simulink model "kalman_at_20_hz"  (R2013b)
settings: Solver=FixedStepDiscrete  StartTime=10  StopTime=250  FixedStep=0.05  RelTol=1e-3
settings Model: Creator=Franta  LastModifiedBy=Franta

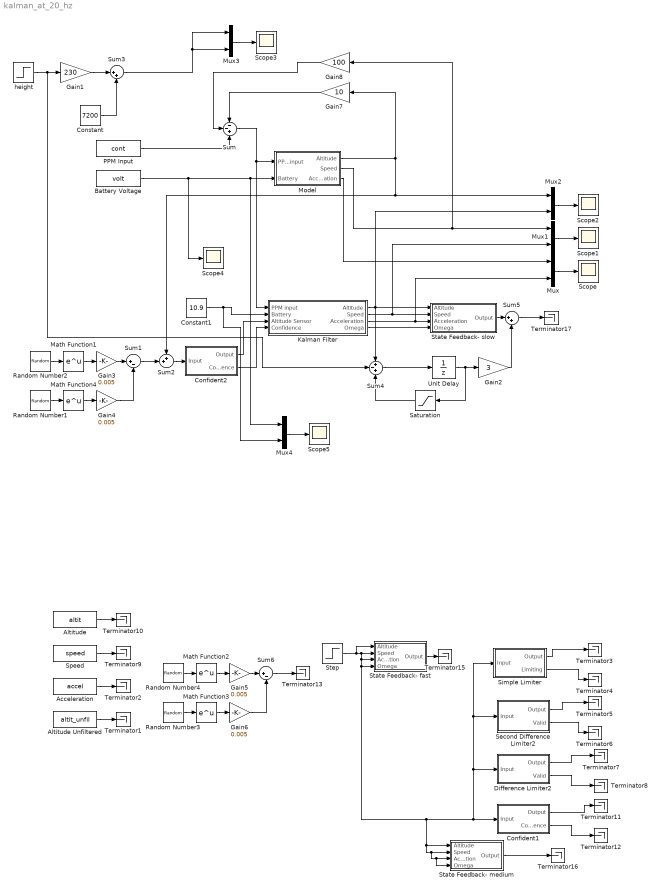
== system kalman_at_20_hz ==
  Acceleration : FromWorkspace  VariableName=accel  SampleTime=0  OutputAfterFinalValue=Holding final value
  Altitude : FromWorkspace  VariableName=altit  SampleTime=0  OutputAfterFinalValue=Holding final value
  Altitude Unfiltered : FromWorkspace  VariableName=altit_unfil  SampleTime=0  OutputAfterFinalValue=Holding final value
  Battery Voltage : FromWorkspace  VariableName=volt  SampleTime=0  OutputAfterFinalValue=Holding final value
  Confident1 : Subsystem
  Confident2 : Subsystem
  Constant : Constant  Value=7200
  Constant1 : Constant  Value=10.9
  Difference Limiter2 : Subsystem
  Gain1 : Gain  Gain=230
  Gain2 : Gain  Gain=3
  Gain{3..6} (4 alike) : Gain  Gain=0.005
  Gain7 : Gain  Gain=10
  Gain8 : Gain  Gain=100
  Kalman Filter : Subsystem
  Math Function{1..4} (4 alike) : Math  SaturateOnIntegerOverflow=on
  Model : Subsystem
  Mux{,1..4} (5 alike) : Mux  Inputs=2
  PPM Input : FromWorkspace  VariableName=cont  SampleTime=0  OutputAfterFinalValue=Holding final value
  Random Number1 : RandomNumber  Variance=4  Seed=1  SampleTime=0.05
  Random Number2 : RandomNumber  Variance=4  SampleTime=0.05
  Random Number3 : RandomNumber  Variance=4  Seed=1  SampleTime=0.05
  Random Number4 : RandomNumber  Variance=4  SampleTime=0.05
  Saturation : Saturate  UpperLimit=100  LowerLimit=-100
  Scope{,1..5} (6 alike) : Scope
      Scope settings: YMin=0  YMax=47.5
      Scope1 settings: TimeRange=50
      Scope2 settings: SaveName=ScopeData2
      Scope3 settings: SaveName=ScopeData3
      Scope4 settings: SaveName=ScopeData4
      Scope5 settings: SaveName=ScopeData5
  Second Difference Limiter2 : Subsystem
  Simple Limiter : Subsystem
  Speed : FromWorkspace  VariableName=speed  SampleTime=0  OutputAfterFinalValue=Holding final value
  State Feedback- fast : Subsystem
  State Feedback- medium : Subsystem
  State Feedback- slow : Subsystem
  Step : Step  Time=150  SampleTime=0
  Sum : Sum  Inputs=--+
  Sum1 : Sum  Inputs=|+-
  Sum2 : Sum  Inputs=++|
  Sum3 : Sum  Inputs=|++
  Sum4 : Sum  Inputs=+-+
  Sum5 : Sum  Inputs=|++
  Sum6 : Sum  Inputs=|+-
  Terminator{1..13,15..17} (16 alike) : Terminator
  Unit Delay : UnitDelay  SampleTime=-1
  height : Step  Time=225  SampleTime=0
  wires:
  Mux/1 -> Scope/1
  Mux1/1 -> Scope1/1
  Mux2/1 -> Scope2/1
  Battery Voltage/1 -> Scope4/1, Mux4/1, Model/2(Battery)
  Kalman Filter/3(Acceleration) -> Mux/2, State Feedback- slow/3(Acceleration)
  Simple Limiter/1(Output) -> Terminator3/1
  Simple Limiter/2(Limiting) -> Terminator4/1
  Second Difference Limiter2/1(Output) -> Terminator5/1
  Second Difference Limiter2/2(Valid) -> Terminator6/1
  Difference Limiter2/1(Output) -> Terminator7/1
  Difference Limiter2/2(Valid) -> Terminator8/1
  Kalman Filter/1(Altitude) -> Mux2/2, State Feedback- slow/1(Altitude), Sum4/1
  Kalman Filter/2(Speed) -> Mux1/2, State Feedback- slow/2(Speed)
  Confident1/1(Output) -> Terminator11/1
  Confident1/2(Confidence) -> Terminator12/1
  Confident2/1(Output) -> Kalman Filter/3(Altitude Sensor)
  Confident2/2(Confidence) -> Kalman Filter/4(Confidence)
  Mux3/1 -> Scope3/1
  height/1 -> Sum4/2, Gain1/1
  Gain1/1 -> Sum3/1
  Constant/1 -> Sum3/2
  Step/1 -> State Feedback- fast/3(Acceleration), State Feedback- fast/4(Omega), State Feedback- medium/4(Omega), State Feedback- medium/3(Acceleration), State Feedback- medium/2(Speed), State Feedback- medium/1(Altitude), Simple Limiter/1(Input), Second Difference Limiter2/1(Input), Difference Limiter2/1(Input), Confident1/1(Input), State Feedback- fast/2(Speed), State Feedback- fast/1(Altitude)
  Sum4/1 -> Unit Delay/1
  State Feedback- medium/1(Output) -> Terminator16/1
  Unit Delay/1 -> Gain2/1, Saturation/1
  Gain2/1 -> Sum5/2
  State Feedback- slow/1(Output) -> Sum5/1
  State Feedback- fast/1(Output) -> Terminator15/1
  Kalman Filter/4(Omega) -> State Feedback- slow/4(Omega)
  Model/1(Altitude) -> Gain7/1, Mux2/1, Sum2/1
  Model/2(Speed) -> Gain8/1, Mux1/1
  Model/3(Acceleration) -> Mux/1
  Altitude Unfiltered/1 -> Terminator1/1
  Sum2/1 -> Confident2/1(Input)
  Sum1/1 -> Sum2/2
  Random Number4/1 -> Math Function2/1
  Math Function2/1 -> Gain5/1
  Random Number3/1 -> Math Function3/1
  Math Function3/1 -> Gain6/1
  Gain6/1 -> Sum6/2
  Gain5/1 -> Sum6/1
  Sum6/1 -> Terminator13/1
  Acceleration/1 -> Terminator2/1
  Speed/1 -> Terminator9/1
  Altitude/1 -> Terminator10/1
  Random Number2/1 -> Math Function1/1
  Math Function1/1 -> Gain3/1
  Random Number1/1 -> Math Function4/1
  Math Function4/1 -> Gain4/1
  Gain4/1 -> Sum1/2
  Gain3/1 -> Sum1/1
  Saturation/1 -> Sum4/3
  Sum5/1 -> Terminator17/1
  Sum3/1 -> Mux3/2, Mux3/1
  Sum/1 -> Kalman Filter/1(PPM input), Model/1(PPM input)
  Gain7/1 -> Sum/1
  PPM Input/1 -> Sum/3
  Gain8/1 -> Sum/2
  Constant1/1 -> Mux4/2, Kalman Filter/2(Battery)
  Mux4/1 -> Scope5/1

== system kalman_at_20_hz/Confident1 ==
  Input : Inport
  MATLAB Function : MATLAB Function  TreatAsAtomicUnit=on
  Threshold : Constant  Value=0.35
  Unit Delay : UnitDelay  InitialCondition=0.5  SampleTime=-1
  Unit Delay1 : UnitDelay  SampleTime=-1
  Output : Outport
  Confidence : Outport  Port=2
  wires:
  Unit Delay1/1 -> MATLAB Function/4(cycles)
  MATLAB Function/3(cyclesBlind) -> Unit Delay1/1
  MATLAB Function/2(confidence) -> Confidence/1
  Unit Delay/1 -> MATLAB Function/3(lastGood)
  MATLAB Function/1(good) -> Unit Delay/1
  Threshold/1 -> MATLAB Function/2(threshold)
  Input/1 -> MATLAB Function/1(input), Output/1

== system kalman_at_20_hz/Confident2 ==
  Input : Inport
  MATLAB Function : MATLAB Function  TreatAsAtomicUnit=on
  Threshold : Constant  Value=0.35
  Unit Delay : UnitDelay  InitialCondition=0.5  SampleTime=-1
  Unit Delay1 : UnitDelay  SampleTime=-1
  Output : Outport
  Confidence : Outport  Port=2
  wires:
  Input/1 -> Output/1, MATLAB Function/1(input)
  Threshold/1 -> MATLAB Function/2(threshold)
  MATLAB Function/1(good) -> Unit Delay/1
  Unit Delay/1 -> MATLAB Function/3(lastGood)
  MATLAB Function/2(confidence) -> Confidence/1
  MATLAB Function/3(cyclesBlind) -> Unit Delay1/1
  Unit Delay1/1 -> MATLAB Function/4(cycles)

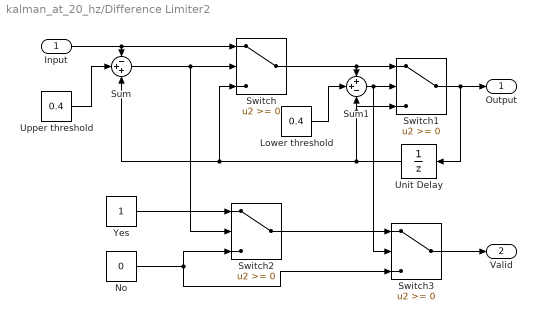
== system kalman_at_20_hz/Difference Limiter2 ==
  Input : Inport
  Lower threshold : Constant  Value=0.4
  No : Constant  Value=0
  Sum : Sum  Inputs=-++
  Sum1 : Sum  Inputs=++-
  Switch{,1..3} (4 alike) : Switch
  Unit Delay : UnitDelay  InitialCondition=1  SampleTime=-1
  Upper threshold : Constant  Value=0.4
  Yes : Constant
  Output : Outport
  Valid : Outport  Port=2
  wires:
  Lower threshold/1 -> Sum1/2
  Switch/1 -> Switch1/1, Sum1/1
  Switch1/1 -> Unit Delay/1, Output/1
  Upper threshold/1 -> Sum/2
  Input/1 -> Switch/1, Sum/1
  Unit Delay/1 -> Sum/3, Switch/3, Switch1/3, Sum1/3
  Sum/1 -> Switch2/2, Switch/2
  Sum1/1 -> Switch3/2, Switch1/2
  Yes/1 -> Switch2/1
  No/1 -> Switch2/3, Switch3/3
  Switch2/1 -> Switch3/1
  Switch3/1 -> Valid/1

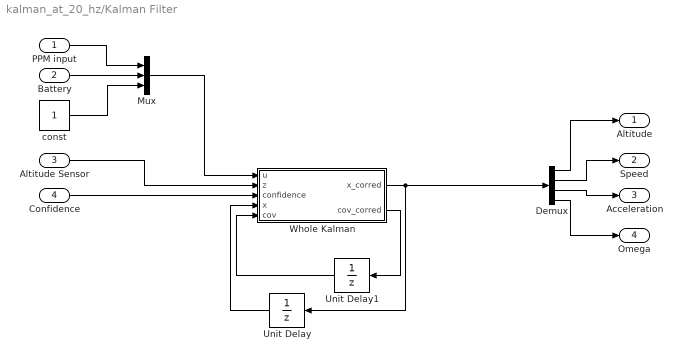
== system kalman_at_20_hz/Kalman Filter ==
  PPM input : Inport
  Battery : Inport  Port=2
  Altitude Sensor : Inport  Port=3
  Confidence : Inport  Port=4
  Demux : Demux
  Mux : Mux  Inputs=3
  Unit Delay : UnitDelay  InitialCondition=[0 0 0 0]'  SampleTime=-1
  Unit Delay1 : UnitDelay  InitialCondition=[1 0 0 0; 0 1 0 0; 0 0 1 0; 0 0 0 1]  SampleTime=-1
  Whole Kalman : MATLAB Function  TreatAsAtomicUnit=on
  const : Constant
  Altitude : Outport
  Speed : Outport  Port=2
  Acceleration : Outport  Port=3
  Omega : Outport  Port=4
  wires:
  Whole Kalman/1(x_corred) -> Demux/1, Unit Delay/1
  Mux/1 -> Whole Kalman/1(u)
  PPM input/1 -> Mux/1
  Battery/1 -> Mux/2
  const/1 -> Mux/3
  Demux/2 -> Speed/1
  Demux/3 -> Acceleration/1
  Demux/1 -> Altitude/1
  Demux/4 -> Omega/1
  Unit Delay1/1 -> Whole Kalman/5(cov)
  Whole Kalman/2(cov_corred) -> Unit Delay1/1
  Unit Delay/1 -> Whole Kalman/4(x)
  Confidence/1 -> Whole Kalman/3(confidence)
  Altitude Sensor/1 -> Whole Kalman/2(z)

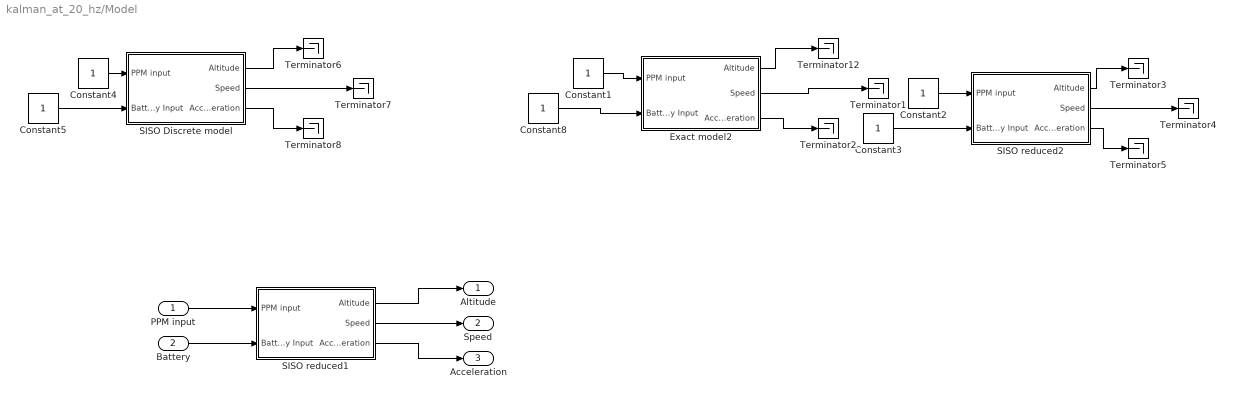
== system kalman_at_20_hz/Model ==
  PPM input : Inport
  Battery : Inport  Port=2
  Constant{1..5,8} (6 alike) : Constant
  Exact model2 : Subsystem
  SISO Discrete model : Subsystem
  SISO reduced1 : Subsystem
  SISO reduced2 : Subsystem
  Terminator{1..8,12} (9 alike) : Terminator
  Altitude : Outport
  Speed : Outport  Port=2
  Acceleration : Outport  Port=3
  wires:
  SISO reduced2/1(Altitude) -> Terminator3/1
  SISO reduced2/2(Speed) -> Terminator4/1
  SISO reduced2/3(Acceleration) -> Terminator5/1
  Constant3/1 -> SISO reduced2/2(Battery Input)
  Constant2/1 -> SISO reduced2/1(PPM input)
  SISO Discrete model/1(Altitude) -> Terminator6/1
  SISO Discrete model/2(Speed) -> Terminator7/1
  SISO Discrete model/3(Acceleration) -> Terminator8/1
  Constant5/1 -> SISO Discrete model/2(Battery Input)
  Constant4/1 -> SISO Discrete model/1(PPM input)
  Constant8/1 -> Exact model2/2(Battery Input)
  Constant1/1 -> Exact model2/1(PPM input)
  Exact model2/1(Altitude) -> Terminator12/1
  Exact model2/2(Speed) -> Terminator1/1
  Exact model2/3(Acceleration) -> Terminator2/1
  PPM input/1 -> SISO reduced1/1(PPM input)
  Battery/1 -> SISO reduced1/2(Battery Input)
  SISO reduced1/1(Altitude) -> Altitude/1
  SISO reduced1/2(Speed) -> Speed/1
  SISO reduced1/3(Acceleration) -> Acceleration/1

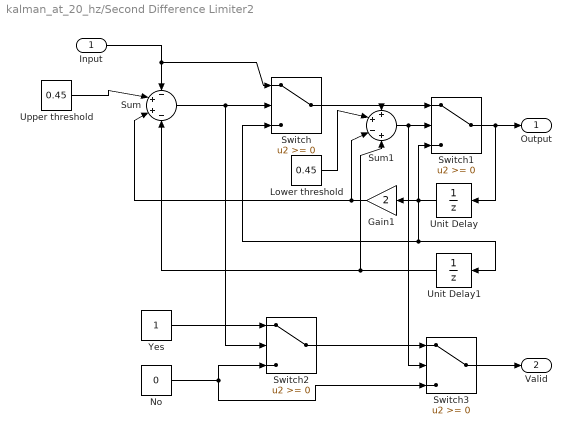
== system kalman_at_20_hz/Second Difference Limiter2 ==
  Input : Inport
  Gain1 : Gain  Gain=2
  Lower threshold : Constant  Value=0.45
  No : Constant  Value=0
  Sum : Sum  Inputs=-++-
  Sum1 : Sum  Inputs=++-+
  Switch{,1..3} (4 alike) : Switch
  Unit Delay : UnitDelay  InitialCondition=1  SampleTime=-1
  Unit Delay1 : UnitDelay  InitialCondition=1  SampleTime=-1
  Upper threshold : Constant  Value=0.45
  Yes : Constant
  Output : Outport
  Valid : Outport  Port=2
  wires:
  Gain1/1 -> Sum1/3, Sum/3
  Switch3/1 -> Valid/1
  Switch2/1 -> Switch3/1
  No/1 -> Switch3/3, Switch2/3
  Yes/1 -> Switch2/1
  Sum1/1 -> Switch1/2, Switch3/2
  Sum/1 -> Switch2/2, Switch/2
  Unit Delay/1 -> Gain1/1, Switch1/3, Unit Delay1/1, Switch/3
  Input/1 -> Switch/1, Sum/1
  Upper threshold/1 -> Sum/2
  Switch1/1 -> Output/1, Unit Delay/1
  Switch/1 -> Switch1/1, Sum1/1
  Lower threshold/1 -> Sum1/2
  Unit Delay1/1 -> Sum1/4, Sum/4

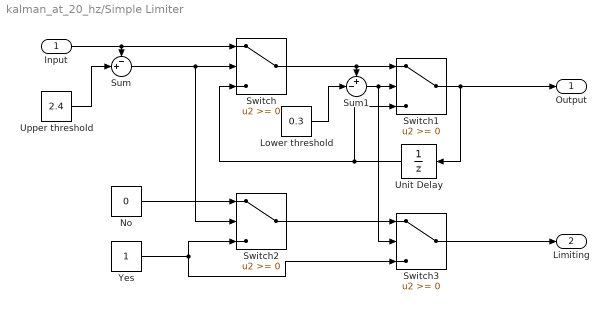
== system kalman_at_20_hz/Simple Limiter ==
  Input : Inport
  Lower threshold : Constant  Value=0.3
  No : Constant  Value=0
  Sum : Sum  Inputs=-+|
  Sum1 : Sum  Inputs=+-|
  Switch{,1..3} (4 alike) : Switch
  Unit Delay : UnitDelay  SampleTime=-1
  Upper threshold : Constant  Value=2.4
  Yes : Constant
  Output : Outport
  Limiting : Outport  Port=2
  wires:
  Unit Delay/1 -> Switch1/3, Switch/3
  Sum/1 -> Switch2/2, Switch/2
  Input/1 -> Sum/1, Switch/1
  Upper threshold/1 -> Sum/2
  Switch1/1 -> Output/1, Unit Delay/1
  Sum1/1 -> Switch3/2, Switch1/2
  Switch/1 -> Sum1/1, Switch1/1
  Lower threshold/1 -> Sum1/2
  No/1 -> Switch2/1
  Yes/1 -> Switch2/3, Switch3/3
  Switch2/1 -> Switch3/1
  Switch3/1 -> Limiting/1

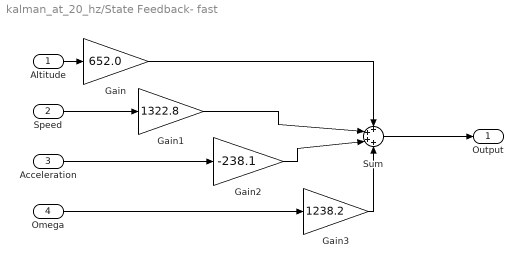
== system kalman_at_20_hz/State Feedback- fast ==
  Altitude : Inport
  Speed : Inport  Port=2
  Acceleration : Inport  Port=3
  Omega : Inport  Port=4
  Gain : Gain  Gain=652.0
  Gain1 : Gain  Gain=1322.8
  Gain2 : Gain  Gain=-238.1
  Gain3 : Gain  Gain=1238.2
  Sum : Sum  Inputs=++++
  Output : Outport
  wires:
  Altitude/1 -> Gain/1
  Speed/1 -> Gain1/1
  Acceleration/1 -> Gain2/1
  Omega/1 -> Gain3/1
  Gain/1 -> Sum/1
  Gain1/1 -> Sum/2
  Gain2/1 -> Sum/3
  Gain3/1 -> Sum/4
  Sum/1 -> Output/1

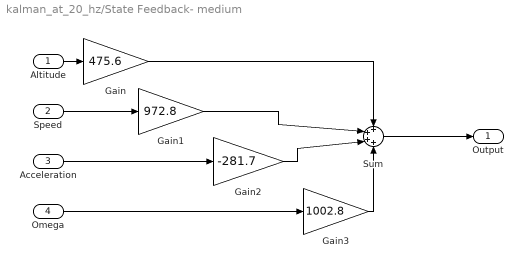
== system kalman_at_20_hz/State Feedback- medium ==
  Altitude : Inport
  Speed : Inport  Port=2
  Acceleration : Inport  Port=3
  Omega : Inport  Port=4
  Gain : Gain  Gain=475.6
  Gain1 : Gain  Gain=972.8
  Gain2 : Gain  Gain=-281.7
  Gain3 : Gain  Gain=1002.8
  Sum : Sum  Inputs=++++
  Output : Outport
  wires:
  Sum/1 -> Output/1
  Gain3/1 -> Sum/4
  Gain2/1 -> Sum/3
  Gain1/1 -> Sum/2
  Gain/1 -> Sum/1
  Omega/1 -> Gain3/1
  Acceleration/1 -> Gain2/1
  Speed/1 -> Gain1/1
  Altitude/1 -> Gain/1

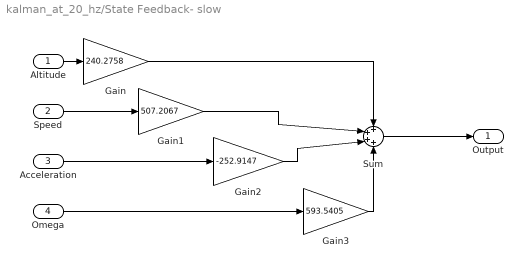
== system kalman_at_20_hz/State Feedback- slow ==
  Altitude : Inport
  Speed : Inport  Port=2
  Acceleration : Inport  Port=3
  Omega : Inport  Port=4
  Gain : Gain  Gain=240.2758
  Gain1 : Gain  Gain=507.2067
  Gain2 : Gain  Gain=-252.9147
  Gain3 : Gain  Gain=593.5405
  Sum : Sum  Inputs=++++
  Output : Outport
  wires:
  Altitude/1 -> Gain/1
  Speed/1 -> Gain1/1
  Acceleration/1 -> Gain2/1
  Omega/1 -> Gain3/1
  Gain/1 -> Sum/1
  Gain1/1 -> Sum/2
  Gain2/1 -> Sum/3
  Gain3/1 -> Sum/4
  Sum/1 -> Output/1

== system kalman_at_20_hz/Model/Exact model2 ==
  PPM input : Inport
  Battery Input : Inport  Port=2
  Demux : Demux
  Discrete State-Space : DiscreteStateSpace  A=[1 0.05 0 0; 0 1 0.05 0; 0 0 0 1; 0 0 -0.65658 1.5714]  B=[0 0 0; 0 0 0; 0.00091141 -0.36830 -2.8005; 0.0011525 -0.052414 -7.5757]  C=[1 0 0 0; 0 1 0 0; 0 0 1 0; 0 0 0 1]  D=[0 0 0; 0 0 0; 0 0 0; 0 0 0]  SampleTime=0.05
  Mux : Mux  Inputs=3
  Terminator : Terminator
  const : Constant
  Altitude : Outport
  Speed : Outport  Port=2
  Acceleration : Outport  Port=3
  wires:
  const/1 -> Mux/3
  Battery Input/1 -> Mux/2
  PPM input/1 -> Mux/1
  Discrete State-Space/1 -> Demux/1
  Demux/3 -> Acceleration/1
  Demux/2 -> Speed/1
  Demux/1 -> Altitude/1
  Mux/1 -> Discrete State-Space/1
  Demux/4 -> Terminator/1

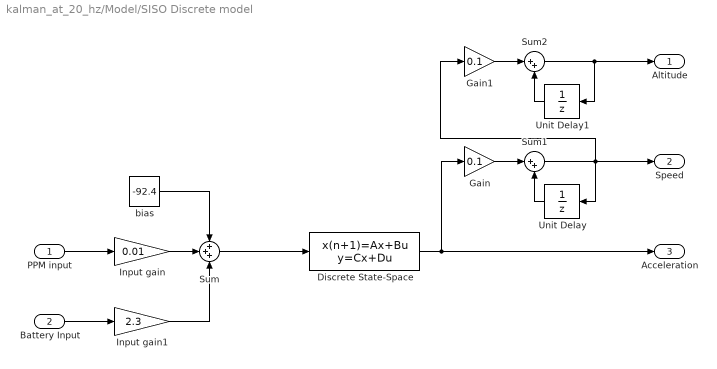
== system kalman_at_20_hz/Model/SISO Discrete model ==
  PPM input : Inport
  Battery Input : Inport  Port=2
  Discrete State-Space : DiscreteStateSpace  A=[0 1; -0.67523 1.64069]  B=[0.28811; 0.18591]  C=[1 0]  D=0  SampleTime=0.1
  Gain : Gain  Gain=0.1
  Gain1 : Gain  Gain=0.1
  Input gain : Gain  Gain=0.01
  Input gain1 : Gain  Gain=2.3
  Sum : Sum  Inputs=+++
  Sum1 : Sum  Inputs=|++
  Sum2 : Sum  Inputs=|++
  Unit Delay : UnitDelay  SampleTime=-1
  Unit Delay1 : UnitDelay  InitialCondition=1  SampleTime=-1
  bias : Constant  Value=-92.4
  Altitude : Outport
  Speed : Outport  Port=2
  Acceleration : Outport  Port=3
  wires:
  PPM input/1 -> Input gain/1
  Battery Input/1 -> Input gain1/1
  Input gain/1 -> Sum/2
  Input gain1/1 -> Sum/3
  bias/1 -> Sum/1
  Sum/1 -> Discrete State-Space/1
  Discrete State-Space/1 -> Gain/1, Acceleration/1
  Unit Delay/1 -> Sum1/2
  Sum1/1 -> Unit Delay/1, Gain1/1, Speed/1
  Sum2/1 -> Unit Delay1/1, Altitude/1
  Unit Delay1/1 -> Sum2/2
  Gain/1 -> Sum1/1
  Gain1/1 -> Sum2/1

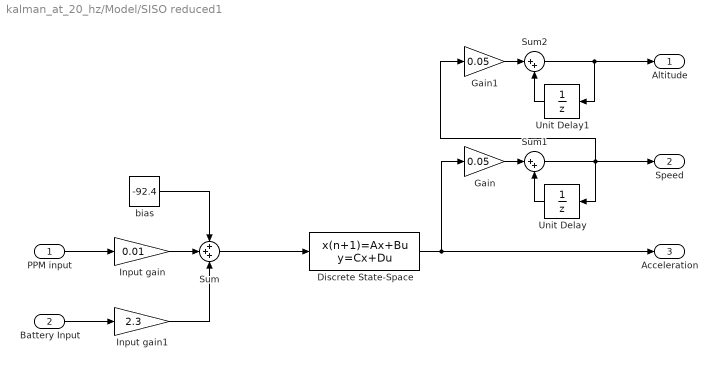
== system kalman_at_20_hz/Model/SISO reduced1 ==
  PPM input : Inport
  Battery Input : Inport  Port=2
  Discrete State-Space : DiscreteStateSpace  A=[0.8379]  B=[0.1382]  C=[1]  D=0  SampleTime=0.05
  Gain : Gain  Gain=0.05
  Gain1 : Gain  Gain=0.05
  Input gain : Gain  Gain=0.01
  Input gain1 : Gain  Gain=2.3
  Sum : Sum  Inputs=+++
  Sum1 : Sum  Inputs=|++
  Sum2 : Sum  Inputs=|++
  Unit Delay : UnitDelay  SampleTime=-1
  Unit Delay1 : UnitDelay  SampleTime=-1
  bias : Constant  Value=-92.4
  Altitude : Outport
  Speed : Outport  Port=2
  Acceleration : Outport  Port=3
  wires:
  PPM input/1 -> Input gain/1
  Battery Input/1 -> Input gain1/1
  Input gain/1 -> Sum/2
  Input gain1/1 -> Sum/3
  bias/1 -> Sum/1
  Sum/1 -> Discrete State-Space/1
  Discrete State-Space/1 -> Gain/1, Acceleration/1
  Unit Delay/1 -> Sum1/2
  Sum1/1 -> Unit Delay/1, Gain1/1, Speed/1
  Sum2/1 -> Unit Delay1/1, Altitude/1
  Unit Delay1/1 -> Sum2/2
  Gain/1 -> Sum1/1
  Gain1/1 -> Sum2/1

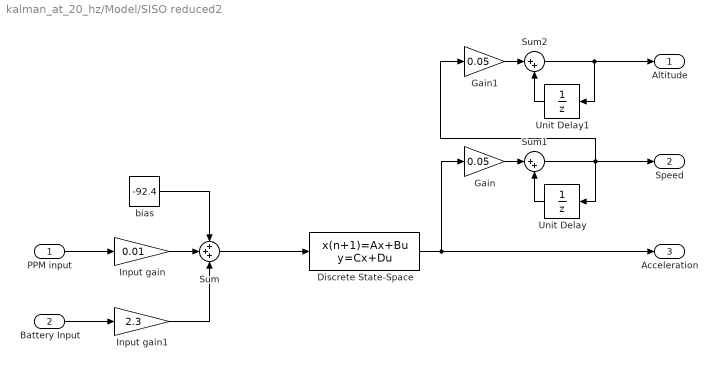
== system kalman_at_20_hz/Model/SISO reduced2 ==
  PPM input : Inport
  Battery Input : Inport  Port=2
  Discrete State-Space : DiscreteStateSpace  A=[0.8379]  B=[0.1382]  C=[1]  D=0  SampleTime=0.05
  Gain : Gain  Gain=0.05
  Gain1 : Gain  Gain=0.05
  Input gain : Gain  Gain=0.01
  Input gain1 : Gain  Gain=2.3
  Sum : Sum  Inputs=+++
  Sum1 : Sum  Inputs=|++
  Sum2 : Sum  Inputs=|++
  Unit Delay : UnitDelay  SampleTime=-1
  Unit Delay1 : UnitDelay  SampleTime=-1
  bias : Constant  Value=-92.4
  Altitude : Outport
  Speed : Outport  Port=2
  Acceleration : Outport  Port=3
  wires:
  Gain1/1 -> Sum2/1
  Gain/1 -> Sum1/1
  Unit Delay1/1 -> Sum2/2
  Sum2/1 -> Altitude/1, Unit Delay1/1
  Sum1/1 -> Speed/1, Gain1/1, Unit Delay/1
  Unit Delay/1 -> Sum1/2
  Discrete State-Space/1 -> Acceleration/1, Gain/1
  Sum/1 -> Discrete State-Space/1
  bias/1 -> Sum/1
  Input gain1/1 -> Sum/3
  Input gain/1 -> Sum/2
  Battery Input/1 -> Input gain1/1
  PPM input/1 -> Input gain/1

== matlab function kalman_at_20_hz/Confident2/MATLAB Function ==
  data: input input; threshold input; good output; lastGood input; confidence output; cycles input; cyclesBlind output
function [good, confidence, cyclesBlind] = confident(input, threshold, lastGood, cycles)

if (input == lastGood)
    good = lastGood;    
    confidence = 1;
    cyclesBlind = 0;
else
    if (abs(input - lastGood) > threshold)
        if (cycles < 16)
            good = lastGood;
            confidence = (2^cycles)/65536;
            cyclesBlind = cycles + 1;
        else
            good = input;
            confidence = 1;
            cyclesBlind = 0;
        end        
    else
        good = input;
        confidence = 1;
        cyclesBlind = 0;
    end
end

== matlab function kalman_at_20_hz/Kalman Filter/Whole Kalman ==
  data: u input; z input; confidence input; x_corred output; cov_corred output; x input; cov input
function [x_corred, cov_corred] = kalman(u, z, confidence, x, cov)
A = [1 0.05 0 0; 0 1 0.05 0; 0 0 0 1; 0 0 -0.65658 1.5714];
B = [0 0 0; 0 0 0; 0.00091141 -0.36830 -2.8005; 0.0011525 -0.052414 -7.5757];
P = [1 0 0 0];
Q = 100/confidence;
R = [1 0 0 0; 0 1 0 0; 0 0 1 0; 0 0 0 1];

%prediction
x_next = A*x + B*u;
cov_next = (A*cov*A') + R;

%correction
if (confidence > 0.001)
    K = (cov_next*P')/((P*cov_next*P') + Q);
    x_corred = x_next + K*(z - P*x_next);
    cov_corred = (eye(4) - K*P)*cov_next;
else
    x_corred = x_next;
    cov_corred = cov_next;
end

== matlab function kalman_at_20_hz/Confident1/MATLAB Function ==
  data: input input; threshold input; good output; lastGood input; confidence output; cycles input; cyclesBlind output
function [good, confidence, cyclesBlind] = confident(input, threshold, lastGood, cycles)

if (input == lastGood)
    good = lastGood;    
    confidence = 0;
    cyclesBlind = 0;
else
    if (abs(input - lastGood) > threshold)
        if (cycles < 16)
            good = lastGood;
            confidence = (2^cycles)/65536;
            cyclesBlind = cycles + 1;
        else
            good = input;
            confidence = 1;
            cyclesBlind = 0;
        end        
    else
        good = input;
        confidence = 1;
        cyclesBlind = 0;
    end
end
